simulink model "serial_5_channels"  (R2015a)
settings: Solver=ode3  StartTime=0.0  StopTime=0.5  FixedStep=0.001  RelTol=1e-3
undefined symbols (not defined in the file or in its folder): LF, serial
libraries: instrumentlib x2
settings Model: Creator=rblan  LastModifiedBy=rblan
settings HardwareCC: ProdBitPerInt=16  ProdBitPerPointer=16  ProdLargestAtomicInteger=Integer  ProdLargestAtomicFloat=Float  ProdIntDivRoundTo=Zero  ProdEndianess=LittleEndian  ProdWordSize=16  ProdHWDeviceType=Microchip->dsPIC

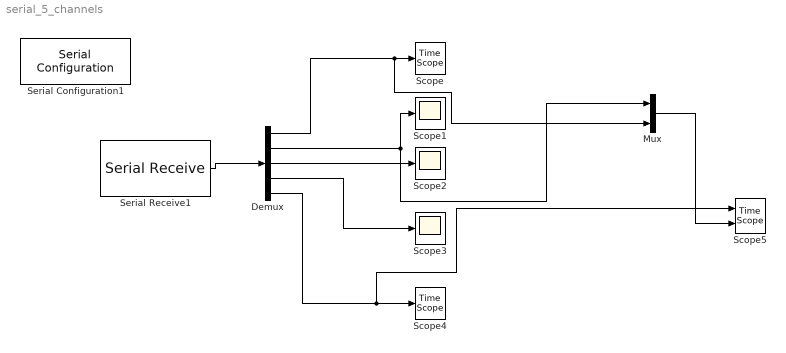
== system serial_5_channels ==
  Demux : Demux  Outputs=5
  Mux : Mux  Inputs=2
  Scope : TimeScope
  Scope1 : Scope
      settings: YMin=-2e+28  YMax=0  DataFormat=Structure
  Scope2 : Scope
      settings: YMin=-2e+28  YMax=0  SaveName=ScopeData2  DataFormat=Structure
  Scope3 : Scope
      settings: YMin=0  YMax=1087.88  SaveName=ScopeData3  DataFormat=Structure
  Scope4 : TimeScope
  Scope5 : TimeScope  NumInputPorts=2
  Serial Configuration1 : instrumentlib/Serial Configuration  Priority=-200000  ComPortMenu=<Please select a port...>  ComPort=COM3  ObjConstructor=serial('COM3');  BaudRate=460800  DataBits=8  Parity=none  StopBits=1  FlowControl=none  Timeout=10  ByteOrder=BigEndian
  Serial Receive1 : instrumentlib/Serial Receive  ComPortMenu=COM3  ComPort=COM3  ObjConstructor=serial('COM3');  Terminator=LF ('\n')  DataSize="[5  1]"  DataType=single  EnableBlockingMode=on  ActionDataUnavailable=Output last received value  CustomValue=0  SampleTime=0.001
  wires:
  Serial Receive1/1 -> Demux/1
  Demux/1 -> Mux/2, Scope/1
  Demux/2 -> Mux/1, Scope1/1
  Demux/3 -> Scope2/1
  Demux/4 -> Scope3/1
  Demux/5 -> Scope5/1, Scope4/1
  Mux/1 -> Scope5/2
